simulink model "Tutorial_Simulink_3"  (R2023b)
settings: Solver=VariableStepAuto  StartTime=0.0  StopTime=10.0  MaxStep=0.05  RelTol=1e-3
settings Model: Creator=admin  LastModifiedBy=admin

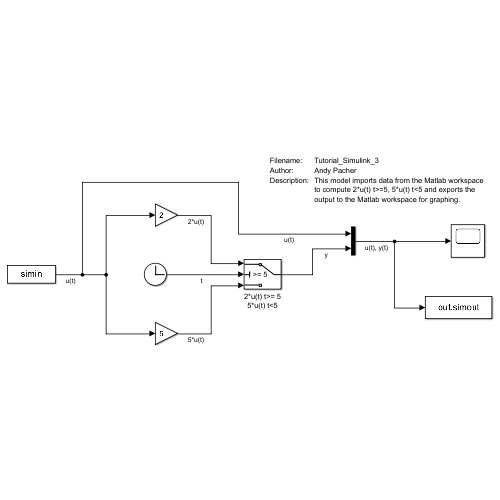
[thumbnail: Simulink's stored preview of the top-level diagram]
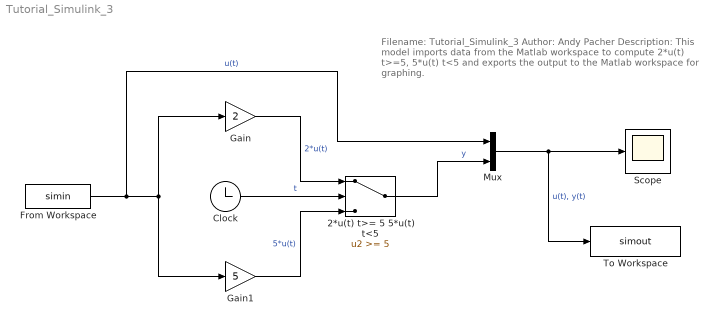
== system Tutorial_Simulink_3 ==
  note: Filename:	Tutorial_Simulink_3
      | Author:		Andy Pacher
      | Description:	This model imports data from the Matlab workspace
      | 			to compute 2*u(t) t>=5, 5*u(t) t<5 and exports the
      | 			output to the Matlab workspace for graphing.
  2*u(t) t>= 5 5*u(t) t<5 : Switch  Threshold=5  SaturateOnIntegerOverflow=off  InputSameDT=off
  Clock : Clock
  From Workspace : FromWorkspace  VariableName=simin
  Gain : Gain  Gain=2
  Gain1 : Gain  Gain=5
  Mux : Mux  Inputs=2
  Scope : Scope
  To Workspace : ToWorkspace  VariableName=simout  SaveFormat=Timeseries  SampleTime=-1
  wires:
  From Workspace/1 -> Mux/1, Gain/1, Gain1/1  "u(t)"
  Clock/1 -> 2*u(t) t>= 5 5*u(t) t<5/2  "t"
  Gain/1 -> 2*u(t) t>= 5 5*u(t) t<5/1  "2*u(t)"
  2*u(t) t>= 5 5*u(t) t<5/1 -> Mux/2  "y"
  Mux/1 -> To Workspace/1, Scope/1  "u(t), y(t)"
  Gain1/1 -> 2*u(t) t>= 5 5*u(t) t<5/3  "5*u(t)"
